simulink subsystem "median5"  (R2021b)
settings: Solver=VariableStepAuto  StartTime=0.0  StopTime=10.0  RelTol=1e-3
settings Model: Creator=dileepan  LastModifiedBy=dileepan

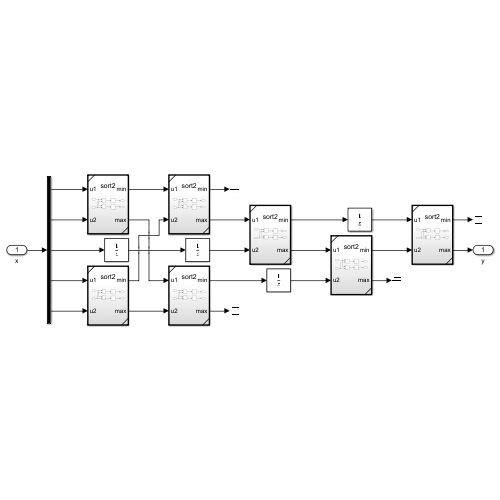
[thumbnail: Simulink's stored preview of the top-level diagram]
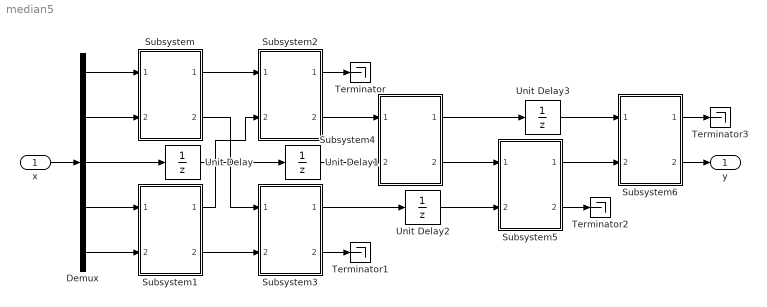
== system median5 ==
  x : Inport
  Demux : Demux  Outputs=5
  Subsystem{,1..6} (7 alike) : Subsystem  TreatAsAtomicUnit=on  ReferencedSubsystem=sort2
  Terminator{,1..3} (4 alike) : Terminator
  Unit Delay{,1..3} (4 alike) : UnitDelay  SampleTime=-1  HasFrameUpgradeWarning=on
  y : Outport
  wires:
  Demux/1 -> Subsystem/1
  Demux/2 -> Subsystem/2
  Demux/4 -> Subsystem1/1
  Demux/5 -> Subsystem1/2
  Demux/3 -> Unit Delay/1
  Subsystem/1 -> Subsystem2/1
  Unit Delay/1 -> Unit Delay1/1
  Subsystem1/2 -> Subsystem3/2
  Subsystem2/2 -> Subsystem4/1
  Unit Delay1/1 -> Subsystem4/2
  Subsystem3/1 -> Unit Delay2/1
  Subsystem/2 -> Subsystem3/1
  Subsystem1/1 -> Subsystem2/2
  x/1 -> Demux/1
  Subsystem4/1 -> Unit Delay3/1
  Subsystem4/2 -> Subsystem5/1
  Unit Delay2/1 -> Subsystem5/2
  Unit Delay3/1 -> Subsystem6/1
  Subsystem5/1 -> Subsystem6/2
  Subsystem6/2 -> y/1
  Subsystem2/1 -> Terminator/1
  Subsystem3/2 -> Terminator1/1
  Subsystem5/2 -> Terminator2/1
  Subsystem6/1 -> Terminator3/1
